simulink model "extended_estimator_2"  (R2024b)
settings: Solver=VariableStepAuto  StartTime=0.0  StopTime=10.0  RelTol=1e-3
undefined symbols (not defined in the file or in its folder): A, A_obs, B, B_obs, C, C_obs, C_rho, D, D_obs, k_c, step_response
settings Model: Creator=andre  LastModifiedBy=andre

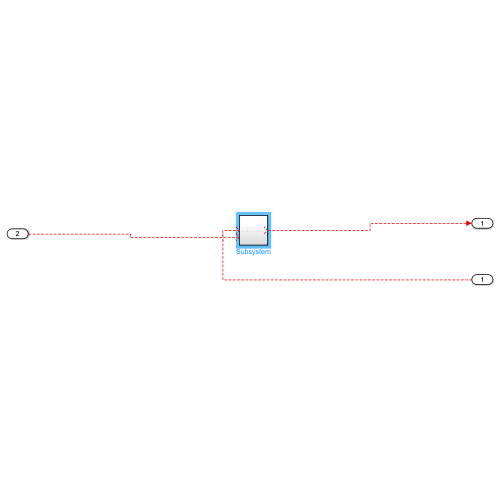
[thumbnail: Simulink's stored preview of the top-level diagram]
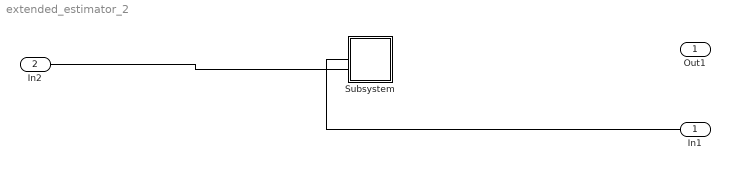
== system extended_estimator_2 ==
  In1 : Inport
  In2 : Inport  Port=2
  Subsystem : Subsystem
  Out1 : Outport
  wires:
  In1/1 -> ?
  In2/1 -> ?
  ? -> Out1/1

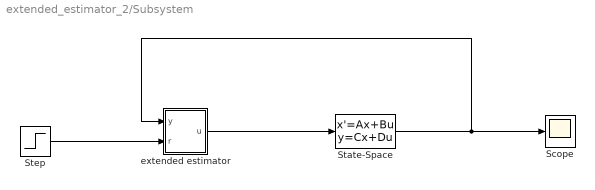
== system extended_estimator_2/Subsystem ==
  Scope : Scope
  State-Space : StateSpace  A=A  B=B  C=C  D=D  InitialCondition=0
  Step : Step  Time=0  After=step_response  SampleTime=0
  extended estimator : Subsystem
  wires:
  extended estimator/1(u) -> State-Space/1
  State-Space/1 -> extended estimator/1(y), Scope/1
  Step/1 -> extended estimator/2(r)

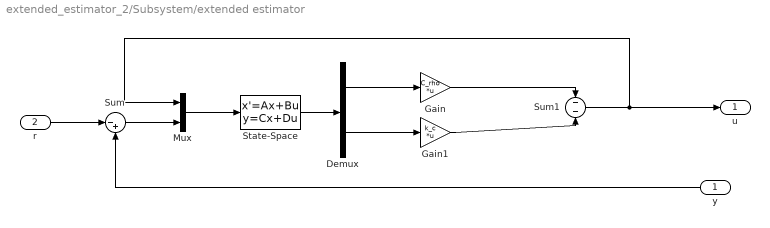
== system extended_estimator_2/Subsystem/extended estimator ==
  y : Inport
  r : Inport  Port=2
  Demux : Demux  Outputs=2
  Gain : Gain  Gain=C_rho  Multiplication=Matrix(K*u)
  Gain1 : Gain  Gain=k_c  Multiplication=Matrix(K*u)
  Mux : Mux  Inputs=2
  State-Space : StateSpace  A=A_obs  B=B_obs  C=C_obs  D=D_obs  InitialCondition=0
  Sum : Sum  Inputs=|-+
  Sum1 : Sum  Inputs=-|-
  u : Outport
  wires:
  Mux/1 -> State-Space/1
  Sum/1 -> Mux/2
  Demux/1 -> Gain/1
  r/1 -> Sum/1
  Gain1/1 -> Sum1/2
  State-Space/1 -> Demux/1
  Sum1/1 -> u/1, Mux/1
  Demux/2 -> Gain1/1
  y/1 -> Sum/2
  Gain/1 -> Sum1/1
